simulink model "openLoopTestBed_R2019b"  (R2017a)
settings: Solver=ode14x  StartTime=0.0  StopTime=10.0  FixedStep=Ts  MaxStep=0.1  RelTol=1e-3
values from neighbouring files (symbols this model uses):
  Ts = 0.01    [conductOpenLoopTestonVirtualPlant.m]    (also in sineSweepOnVirtualPlant.m = 1/Fs)
settings Model: Creator=pbarooah  LastModifiedBy=austin
settings DataIOCC: ExternalInput=u
settings OptimizationCC: LifeSpan=inf
settings DebuggingCC: SFExecutionAtInitializationDiag=none

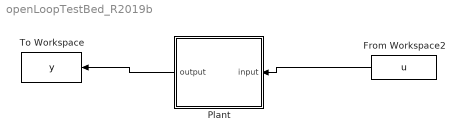
== system openLoopTestBed_R2019b ==
  From Workspace2 : FromWorkspace  VariableName=u  SampleTime=Ts
  "Plant " : Subsystem
  To Workspace : ToWorkspace  VariableName=y  SaveFormat=Structure With Time  SampleTime=Ts
  wires:
  "Plant "/1(output) -> To Workspace/1
  From Workspace2/1 -> "Plant "/1(input)

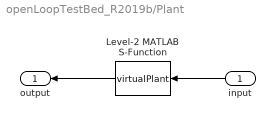
== system openLoopTestBed_R2019b/Plant  ==
  input : Inport
  Level-2 MATLAB S-Function : M-S-Function  FunctionName=virtualPlant
  output : Outport
  wires:
  input/1 -> Level-2 MATLAB S-Function/1
  Level-2 MATLAB S-Function/1 -> output/1
